simulink model "SimFlyback_BF"  (R2014a)
settings: Solver=ode23tb  StartTime=0.0  StopTime=50e-3  FixedStep=11e-6  RelTol=1e-6
libraries: powerlib x12, powerlib_meascontrol x2, simulink x1
settings Model: Creator=hfortin  LastModifiedBy=hugo
settings DataIOCC: SignalLoggingSaveFormat=ModelDataLogs  Refine=4
settings OptimizationCC: ExpressionDepthLimit=2147483647
settings DebuggingCC: UnderspecifiedInitializationDetection=Classic  FcnCallInpInsideContextMsg=UseLocalSettings  StateNameClashWarn=warning
settings GRTTargetCC: CombineOutputUpdateFcns=off  GRTInterface=on

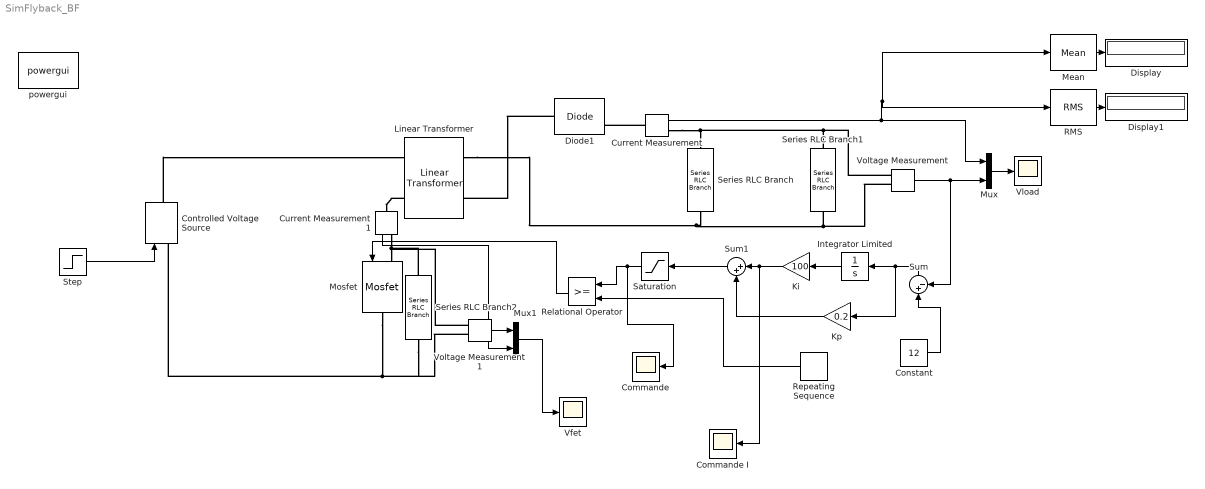
== system SimFlyback_BF ==
  Commande : Scope
      settings: YMin=8.425  YMax=8.975  SaveName=ScopeData3
  Commande I : Scope
      settings: YMin=8.425  YMax=8.975  SaveName=ScopeData4
  Constant : Constant  Value=12
  Controlled Voltage Source : powerlib/Electrical Sources/Controlled Voltage Source  Initialize=off  Source_Type=DC  Amplitude=0  Phase=0  Frequency=0  Measurements=None
  Current Measurement : powerlib/Measurements/Current Measurement  PhasorSimulation=off  OutputType=Complex  PSBequivalent=0
  Current Measurement1 : powerlib/Measurements/Current Measurement  PhasorSimulation=off  OutputType=Complex  PSBequivalent=0
  Diode1 : powerlib/Power Electronics/Diode  Ron=0.001  Lon=0  Vf=0.8  IC=0  UseSnubber=off  Rs=500  Cs=250e-6  Measurements=on
  Display : Display
  Display1 : Display
  Integrator Limited : Integrator  LimitOutput=on  UpperSaturationLimit=1  LowerSaturationLimit=-1
  Ki : Gain  Gain=100
  Kp : Gain  Gain=0.2
  Linear Transformer : powerlib/Elements/Linear Transformer  UNITS=SI  NominalPower=[250e6 60]  winding1=[7.2 0.1 0]  winding2=[1 0.01 0]  ThreeWindings=off  winding3=[3.15e+05 0.7938 0.084225]  RmLm=[1.0805e+6 45.7e-6]  Measurements=None  DataType=on
  Mean : powerlib_meascontrol/Measurements/Mean  Freq=70000  Vinit=0  Ts=0
  Mosfet : powerlib/Power Electronics/Mosfet  Ron=0.01  Lon=0  Rd=0.01  Vfd=0  IC=0  Rs=1e5  Cs=inf  Measurements=off
  Mux : Mux  Inputs=2
  Mux1 : Mux  Inputs=2
  RMS : powerlib_meascontrol/Measurements/RMS  TrueRMS=on  Freq=70000  RMSInit=120  Ts=0
  Relational Operator : RelationalOperator  OutDataTypeStr=boolean
  Repeating Sequence : simulink/Sources/Repeating Sequence  rep_seq_t=[0 1/70000]  rep_seq_y=[0 1]
  Saturation : Saturate  UpperLimit=0.4  LowerLimit=0
  Series RLC Branch : powerlib/Elements/Series RLC Branch  LConnTagsString=__new0  RConnTagsString=__new0  BranchType=C  Resistance=1  Inductance=1e-3  SetiL0=off  InitialCurrent=0  Capacitance=250e-6  Setx0=off  InitialVoltage=10  Measurements=None
  Series RLC Branch1 : powerlib/Elements/Series RLC Branch  LConnTagsString=__new0  RConnTagsString=__new0  BranchType=R  Resistance=0.72  Inductance=1e-3  SetiL0=off  InitialCurrent=0  Capacitance=1e-6  Setx0=off  InitialVoltage=0  Measurements=None
  Series RLC Branch2 : powerlib/Elements/Series RLC Branch  LConnTagsString=__new0  RConnTagsString=__new0  BranchType=RC  Resistance=1000  Inductance=1e-3  SetiL0=off  InitialCurrent=0  Capacitance=10e-6  Setx0=off  InitialVoltage=0  Measurements=None
  Step : Step  Time=30e-3  Before=100  After=150  SampleTime=0
  Sum : Sum  Inputs=|+-
  Sum1 : Sum  Inputs=|++
  "Vfet " : Scope
      settings: YMin=-25  YMax=250
  Vload : Scope
      settings: TimeRange=0.05  YMin=11.1  YMax=12.1
  Voltage Measurement : powerlib/Measurements/Voltage Measurement  PhasorSimulation=off  OutputType=Complex  PSBequivalent=0
  Voltage Measurement1 : powerlib/Measurements/Voltage Measurement  PhasorSimulation=off  OutputType=Complex  PSBequivalent=0
  powergui : powerlib/powergui  Priority=1  SimulationMode=Continuous  SolverType=Tustin  SampleTime=11e-6  frequency=60  SPID=off  DisableSnubberDevices=off  DisableRonSwitches=off  DisableVfSwitches=off  SwTol=0  Interpol=off  DisplayEquations=off  Ts=0  methode=off  frequencyindice=0  Pbase=100e6  ErrMax=1e-4  Iterations=50  UnitsV=kV  UnitsW=MW  FunctionMessages=off  echomessages=off  HookPort=off  EnableUseOfTLC=off  x0status=blocks  RestoreLinks=warning  ResistiveCurrentMeasurement=off  Frange=[0:2:500]  Ylog=off  Xlog=on  ShowGrid=off  save=off  variable=ZData  structure=0  ZoomFFT=on  StartTime=0.0  cycles=1  DisplayStyle=1  fundamental=60  FreqAxis=off  MaxFrequency=1000  frequencyindicesteady=1  RmsSteady=1  display=off
  wires:
  Voltage Measurement/1 -> Mux/2, Sum/2
  Constant/1 -> Sum/1
  Sum/1 -> Kp/1, Integrator Limited/1
  Integrator Limited/1 -> Ki/1
  Ki/1 -> Commande I/1, Sum1/1
  Kp/1 -> Sum1/2
  Repeating Sequence/1 -> Relational Operator/2
  Relational Operator/1 -> Mosfet/1
  Sum1/1 -> Saturation/1
  Saturation/1 -> Commande/1, Relational Operator/1
  Step/1 -> Controlled Voltage Source/1
  Current Measurement/1 -> Mean/1, RMS/1, Mux/1
  Mux/1 -> Vload/1
  Mux1/1 -> "Vfet "/1
  Voltage Measurement1/1 -> Mux1/1
  Current Measurement1/1 -> Mux1/2
  Mean/1 -> Display/1
  RMS/1 -> Display1/1
  connections:
  Series RLC Branch2/LConn1 -- Voltage Measurement1/LConn1 -- Current Measurement1/RConn1 -- Mosfet/LConn1
  Mosfet/RConn1 -- Controlled Voltage Source/LConn1 -- Series RLC Branch2/RConn1 -- Voltage Measurement1/LConn2
  Series RLC Branch/RConn1 -- Linear Transformer/RConn1 -- Voltage Measurement/LConn2 -- Series RLC Branch1/RConn1
  Controlled Voltage Source/RConn1 -- Linear Transformer/LConn1
  Series RLC Branch1/LConn1 -- Voltage Measurement/LConn1 -- Current Measurement/RConn1 -- Series RLC Branch/LConn1
  Diode1/LConn1 -- Linear Transformer/RConn2
  Current Measurement/LConn1 -- Diode1/RConn1
  Linear Transformer/LConn2 -- Current Measurement1/LConn1
